simulink model "tb"  (R2023a)
settings: Solver=VariableStepAuto  StartTime=0.0  StopTime=10.0  RelTol=1e-3
libraries: simulink x2
settings Model: Creator=Francesco  LastModifiedBy=Francesco

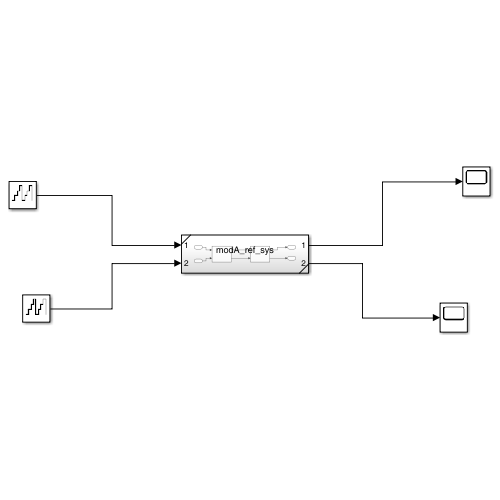
[thumbnail: Simulink's stored preview of the top-level diagram]
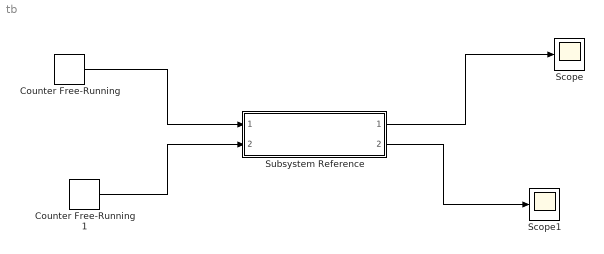
== system tb ==
  Counter Free-Running : simulink/Sources/Counter Free-Running  NumBits=16  tsamp=-1
  Counter Free-Running1 : simulink/Sources/Counter Free-Running  NumBits=16  tsamp=-1
  Scope : Scope
  Scope1 : Scope
  Subsystem Reference : Subsystem  ReferencedSubsystem=modA_ref_sys
  wires:
  Counter Free-Running/1 -> Subsystem Reference/1
  Counter Free-Running1/1 -> Subsystem Reference/2
  Subsystem Reference/1 -> Scope/1
  Subsystem Reference/2 -> Scope1/1
